simulink model "Self_Balancing"  (R2017a)
settings: Solver=VariableStepAuto  StartTime=0.0  StopTime=10.0  RelTol=1e-3
settings Model: Creator=Administrator  LastModifiedBy=Administrator

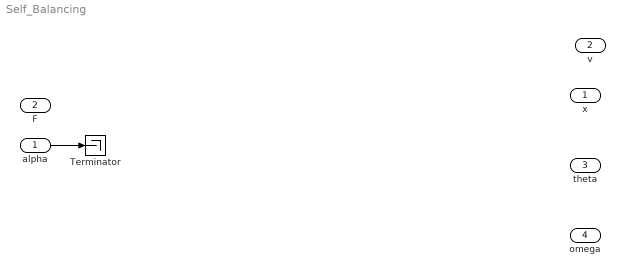
== system Self_Balancing ==
  alpha : Inport
  F : Inport  Port=2
  Terminator : Terminator
  x : Outport
  v : Outport  Port=2
  theta : Outport  Port=3
  omega : Outport  Port=4
  wires:
  alpha/1 -> Terminator/1
  ? -> v/1  "x'"
